simulink model "lwr_scheme_acc"  (R2024a)
settings: Solver=ode15s  StartTime=0.0  StopTime=10.0  FixedStep=0.1  RelTol=1e-3
undefined symbols (not defined in the file): X, Y, Z
libraries: sm_lib x73, nesl_utility x22, robotmaniplib x9, dspinverses x6
(part 2 of 2)

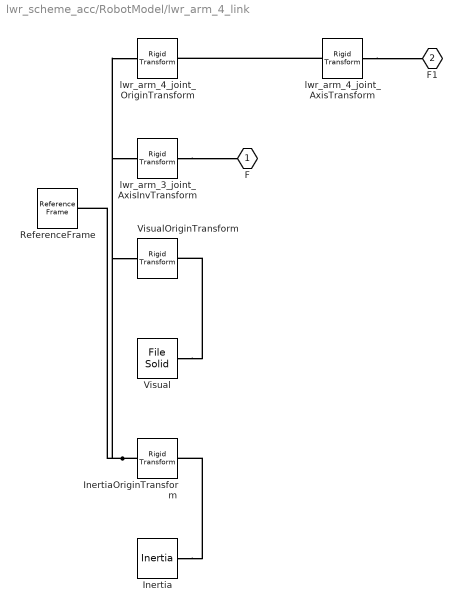
== system lwr_scheme_acc/RobotModel/lwr_arm_4_link ==
  Inertia : sm_lib/Body Elements/Inertia  InertiaType=Custom  Mass=2  MassUnits=kg  CenterOfMass=[0, 0, 0]  CenterOfMassUnits=m  MomentsOfInertia=[0.0136666666667, 0.0118666666667, 0.003000000000000001]  MomentsOfInertiaUnits=kg*m^2  ProductsOfInertia=[0, 0, 0]  ProductsOfInertiaUnits=kg*m^2  GraphicType=None  MarkerShape=Inertia  MarkerSize=20  GraphicVisPropType=SimpleVisualProperties  GraphicDiffuseColor=[0.5 0.5 0.5]  GraphicOpacity=1  GraphicSpecularColor=[0.5 0.5 0.5 1.0]  GraphicAmbientColor=[0.15 0.15 0.15 1.0]  GraphicEmissiveColor=[0.0 0.0 0.0 1.0]  GraphicShininess=75
  InertiaOriginTransform : sm_lib/Frames and Transforms/Rigid Transform  RotationMethod=RotationSequence  FollAlignAxisA=+X  BaseAlignAxisA=+Y  FollAlignAxisB=+Y  BaseAlignAxisB=+Z  RotationStandardAxis=+Z  RotationAngle=0  RotationAngleUnits=deg  RotationArbitraryAxis=[0 0 1]  RotationSequenceAxes=BaseAxes  RotationSequence=XYZ  RotationSequenceAngles=[0, 0, 0]  RotationSequenceAnglesUnits=rad  RotationMatrix=[1 0 0;0 1 0;0 0 1]  Quaternion=[1 0 0 0]  TranslationMethod=Cartesian  TranslationCartesianOffset=[0, 0.06, 0.07000000000000001]  TranslationCartesianOffsetUnits=m  TranslationStandardAxis=+Z  TranslationStandardOffset=0  TranslationStandardOffsetUnits=m  TranslationROffset=0  TranslationROffsetUnits=m  TranslationThetaOffset=0  TranslationThetaOffsetUnits=deg  TranslationZOffset=0  TranslationZOffsetUnits=m
  ReferenceFrame : sm_lib/Frames and Transforms/Reference Frame
  Visual : sm_lib/Body Elements/File Solid  ExtGeomFileName=/Users/salvatore/Desktop/Università/Development/Rob-HW/Damping-in-the-null-space-for-a-redundant-robot/robot_model/kuka-lwr-4plus/meshes/arm_segment_b.stl  UnitType=Custom  ExtGeomFileUnits=m  StepReaderType=HEX  ExportConvexHullGeometry=off  InertiaType=Custom  BasedOnType=DensityFromFile  Density=1000  DensityUnits=kg/m^3  Mass=0  MassUnits=kg  CenterOfMass=[0, 0, 0]  CenterOfMassUnits=m  MomentsOfInertia=[0, 0, 0]  MomentsOfInertiaUnits=kg*m^2  ProductsOfInertia=[0, 0, 0]  ProductsOfInertiaUnits=kg*m^2  GraphicType=FromGeometry  MarkerShape=Sphere  MarkerSize=10  GraphicVisPropType=SimpleVisualProperties  GraphicDiffuseColor=[1, 0.487, 0]  GraphicOpacity=1  GraphicSpecularColor=[0.5 0.5 0.5 1.0]  GraphicAmbientColor=[0.15 0.15 0.15 1.0]  GraphicEmissiveColor=[0.0 0.0 0.0 1.0]  GraphicShininess=75  DoExposeReferenceFrame=on  SerializedFrames=<Frames/>
  VisualOriginTransform : sm_lib/Frames and Transforms/Rigid Transform  RotationMethod=RotationSequence  FollAlignAxisA=+X  BaseAlignAxisA=+Y  FollAlignAxisB=+Y  BaseAlignAxisB=+Z  RotationStandardAxis=+Z  RotationAngle=0  RotationAngleUnits=deg  RotationArbitraryAxis=[0 0 1]  RotationSequenceAxes=BaseAxes  RotationSequence=XYZ  RotationSequenceAngles=[-3.141592653589793, -2.068231071102144e-13, 2.068231071102144e-13]  RotationSequenceAnglesUnits=rad  RotationMatrix=[1 0 0;0 1 0;0 0 1]  Quaternion=[1 0 0 0]  TranslationMethod=Cartesian  TranslationCartesianOffset=[0, 0, 0.2]  TranslationCartesianOffsetUnits=m  TranslationStandardAxis=+Z  TranslationStandardOffset=0  TranslationStandardOffsetUnits=m  TranslationROffset=0  TranslationROffsetUnits=m  TranslationThetaOffset=0  TranslationThetaOffsetUnits=deg  TranslationZOffset=0  TranslationZOffsetUnits=m
  lwr_arm_3_joint_AxisInvTransform : sm_lib/Frames and Transforms/Rigid Transform  RotationMethod=ArbitraryAxis  FollAlignAxisA=+X  BaseAlignAxisA=+Y  FollAlignAxisB=+Y  BaseAlignAxisB=+Z  RotationStandardAxis=+Z  RotationAngle=1.570796326794897  RotationAngleUnits=rad  RotationArbitraryAxis=[-1, 0, 0]  RotationSequenceAxes=FollowerAxes  RotationSequence=XYX  RotationSequenceAngles=[0 0 0]  RotationSequenceAnglesUnits=deg  RotationMatrix=[1 0 0;0 1 0;0 0 1]  Quaternion=[1 0 0 0]  TranslationMethod=Cartesian  TranslationCartesianOffset=[0, 0, 0]  TranslationCartesianOffsetUnits=m  TranslationStandardAxis=+Z  TranslationStandardOffset=0  TranslationStandardOffsetUnits=m  TranslationROffset=0  TranslationROffsetUnits=m  TranslationThetaOffset=0  TranslationThetaOffsetUnits=deg  TranslationZOffset=0  TranslationZOffsetUnits=m
  lwr_arm_4_joint_AxisTransform : sm_lib/Frames and Transforms/Rigid Transform  RotationMethod=ArbitraryAxis  FollAlignAxisA=+X  BaseAlignAxisA=+Y  FollAlignAxisB=+Y  BaseAlignAxisB=+Z  RotationStandardAxis=+Z  RotationAngle=0  RotationAngleUnits=rad  RotationArbitraryAxis=[1, 0, 0]  RotationSequenceAxes=FollowerAxes  RotationSequence=XYX  RotationSequenceAngles=[0 0 0]  RotationSequenceAnglesUnits=deg  RotationMatrix=[1 0 0;0 1 0;0 0 1]  Quaternion=[1 0 0 0]  TranslationMethod=Cartesian  TranslationCartesianOffset=[0, 0, 0]  TranslationCartesianOffsetUnits=m  TranslationStandardAxis=+Z  TranslationStandardOffset=0  TranslationStandardOffsetUnits=m  TranslationROffset=0  TranslationROffsetUnits=m  TranslationThetaOffset=0  TranslationThetaOffsetUnits=deg  TranslationZOffset=0  TranslationZOffsetUnits=m
  lwr_arm_4_joint_OriginTransform : sm_lib/Frames and Transforms/Rigid Transform  RotationMethod=RotationSequence  FollAlignAxisA=+X  BaseAlignAxisA=+Y  FollAlignAxisB=+Y  BaseAlignAxisB=+Z  RotationStandardAxis=+Z  RotationAngle=0  RotationAngleUnits=deg  RotationArbitraryAxis=[0 0 1]  RotationSequenceAxes=BaseAxes  RotationSequence=XYZ  RotationSequenceAngles=[0, 0, 0]  RotationSequenceAnglesUnits=rad  RotationMatrix=[1 0 0;0 1 0;0 0 1]  Quaternion=[1 0 0 0]  TranslationMethod=Cartesian  TranslationCartesianOffset=[0, 0, 0.2]  TranslationCartesianOffsetUnits=m  TranslationStandardAxis=+Z  TranslationStandardOffset=0  TranslationStandardOffsetUnits=m  TranslationROffset=0  TranslationROffsetUnits=m  TranslationThetaOffset=0  TranslationThetaOffsetUnits=deg  TranslationZOffset=0  TranslationZOffsetUnits=m
  F : PMIOPort  Side=Left
  F1 : PMIOPort  Port=2  Side=Right
  connections:
  Inertia/RConn1 -- InertiaOriginTransform/RConn1
  ReferenceFrame/RConn1 -- InertiaOriginTransform/LConn1 -- VisualOriginTransform/LConn1 -- lwr_arm_3_joint_AxisInvTransform/LConn1 -- lwr_arm_4_joint_OriginTransform/LConn1
  Visual/RConn1 -- VisualOriginTransform/RConn1
  lwr_arm_3_joint_AxisInvTransform/RConn1 -- F/RConn1
  lwr_arm_4_joint_AxisTransform/RConn1 -- F1/RConn1
  lwr_arm_4_joint_AxisTransform/LConn1 -- lwr_arm_4_joint_OriginTransform/RConn1

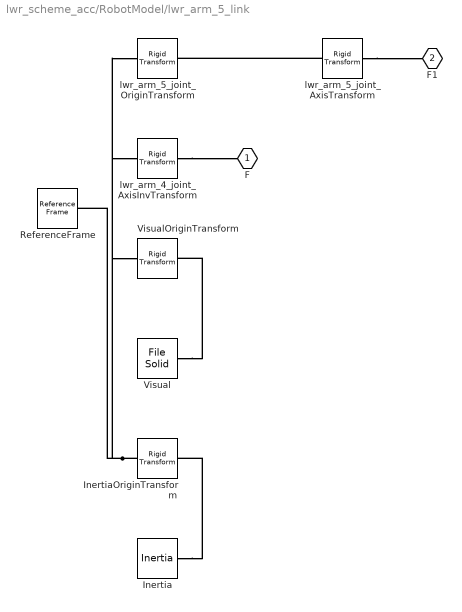
== system lwr_scheme_acc/RobotModel/lwr_arm_5_link ==
  Inertia : sm_lib/Body Elements/Inertia  InertiaType=Custom  Mass=2  MassUnits=kg  CenterOfMass=[0, 0, 0]  CenterOfMassUnits=m  MomentsOfInertia=[0.0126506666667, 0.0108506666667, 0.003]  MomentsOfInertiaUnits=kg*m^2  ProductsOfInertia=[0, 0, 0]  ProductsOfInertiaUnits=kg*m^2  GraphicType=None  MarkerShape=Inertia  MarkerSize=20  GraphicVisPropType=SimpleVisualProperties  GraphicDiffuseColor=[0.5 0.5 0.5]  GraphicOpacity=1  GraphicSpecularColor=[0.5 0.5 0.5 1.0]  GraphicAmbientColor=[0.15 0.15 0.15 1.0]  GraphicEmissiveColor=[0.0 0.0 0.0 1.0]  GraphicShininess=75
  InertiaOriginTransform : sm_lib/Frames and Transforms/Rigid Transform  RotationMethod=RotationSequence  FollAlignAxisA=+X  BaseAlignAxisA=+Y  FollAlignAxisB=+Y  BaseAlignAxisB=+Z  RotationStandardAxis=+Z  RotationAngle=0  RotationAngleUnits=deg  RotationArbitraryAxis=[0 0 1]  RotationSequenceAxes=BaseAxes  RotationSequence=XYZ  RotationSequenceAngles=[0, 0, 0]  RotationSequenceAnglesUnits=rad  RotationMatrix=[1 0 0;0 1 0;0 0 1]  Quaternion=[1 0 0 0]  TranslationMethod=Cartesian  TranslationCartesianOffset=[0, 0, 0.124]  TranslationCartesianOffsetUnits=m  TranslationStandardAxis=+Z  TranslationStandardOffset=0  TranslationStandardOffsetUnits=m  TranslationROffset=0  TranslationROffsetUnits=m  TranslationThetaOffset=0  TranslationThetaOffsetUnits=deg  TranslationZOffset=0  TranslationZOffsetUnits=m
  ReferenceFrame : sm_lib/Frames and Transforms/Reference Frame
  Visual : sm_lib/Body Elements/File Solid  ExtGeomFileName=/Users/salvatore/Desktop/Università/Development/Rob-HW/Damping-in-the-null-space-for-a-redundant-robot/robot_model/kuka-lwr-4plus/meshes/arm_segment_last.stl  UnitType=Custom  ExtGeomFileUnits=m  StepReaderType=HEX  ExportConvexHullGeometry=off  InertiaType=Custom  BasedOnType=DensityFromFile  Density=1000  DensityUnits=kg/m^3  Mass=0  MassUnits=kg  CenterOfMass=[0, 0, 0]  CenterOfMassUnits=m  MomentsOfInertia=[0, 0, 0]  MomentsOfInertiaUnits=kg*m^2  ProductsOfInertia=[0, 0, 0]  ProductsOfInertiaUnits=kg*m^2  GraphicType=FromGeometry  MarkerShape=Sphere  MarkerSize=10  GraphicVisPropType=SimpleVisualProperties  GraphicDiffuseColor=[1, 0.487, 0]  GraphicOpacity=1  GraphicSpecularColor=[0.5 0.5 0.5 1.0]  GraphicAmbientColor=[0.15 0.15 0.15 1.0]  GraphicEmissiveColor=[0.0 0.0 0.0 1.0]  GraphicShininess=75  DoExposeReferenceFrame=on  SerializedFrames=<Frames/>
  VisualOriginTransform : sm_lib/Frames and Transforms/Rigid Transform  RotationMethod=RotationSequence  FollAlignAxisA=+X  BaseAlignAxisA=+Y  FollAlignAxisB=+Y  BaseAlignAxisB=+Z  RotationStandardAxis=+Z  RotationAngle=0  RotationAngleUnits=deg  RotationArbitraryAxis=[0 0 1]  RotationSequenceAxes=BaseAxes  RotationSequence=XYZ  RotationSequenceAngles=[0, 0, -3.141592653589587]  RotationSequenceAnglesUnits=rad  RotationMatrix=[1 0 0;0 1 0;0 0 1]  Quaternion=[1 0 0 0]  TranslationMethod=Cartesian  TranslationCartesianOffset=[0, 0, 0]  TranslationCartesianOffsetUnits=m  TranslationStandardAxis=+Z  TranslationStandardOffset=0  TranslationStandardOffsetUnits=m  TranslationROffset=0  TranslationROffsetUnits=m  TranslationThetaOffset=0  TranslationThetaOffsetUnits=deg  TranslationZOffset=0  TranslationZOffsetUnits=m
  lwr_arm_4_joint_AxisInvTransform : sm_lib/Frames and Transforms/Rigid Transform  RotationMethod=ArbitraryAxis  FollAlignAxisA=+X  BaseAlignAxisA=+Y  FollAlignAxisB=+Y  BaseAlignAxisB=+Z  RotationStandardAxis=+Z  RotationAngle=0  RotationAngleUnits=rad  RotationArbitraryAxis=[1, 0, 0]  RotationSequenceAxes=FollowerAxes  RotationSequence=XYX  RotationSequenceAngles=[0 0 0]  RotationSequenceAnglesUnits=deg  RotationMatrix=[1 0 0;0 1 0;0 0 1]  Quaternion=[1 0 0 0]  TranslationMethod=Cartesian  TranslationCartesianOffset=[0, 0, 0]  TranslationCartesianOffsetUnits=m  TranslationStandardAxis=+Z  TranslationStandardOffset=0  TranslationStandardOffsetUnits=m  TranslationROffset=0  TranslationROffsetUnits=m  TranslationThetaOffset=0  TranslationThetaOffsetUnits=deg  TranslationZOffset=0  TranslationZOffsetUnits=m
  lwr_arm_5_joint_AxisTransform : sm_lib/Frames and Transforms/Rigid Transform  RotationMethod=ArbitraryAxis  FollAlignAxisA=+X  BaseAlignAxisA=+Y  FollAlignAxisB=+Y  BaseAlignAxisB=+Z  RotationStandardAxis=+Z  RotationAngle=1.570796326794897  RotationAngleUnits=rad  RotationArbitraryAxis=[1, 0, 0]  RotationSequenceAxes=FollowerAxes  RotationSequence=XYX  RotationSequenceAngles=[0 0 0]  RotationSequenceAnglesUnits=deg  RotationMatrix=[1 0 0;0 1 0;0 0 1]  Quaternion=[1 0 0 0]  TranslationMethod=Cartesian  TranslationCartesianOffset=[0, 0, 0]  TranslationCartesianOffsetUnits=m  TranslationStandardAxis=+Z  TranslationStandardOffset=0  TranslationStandardOffsetUnits=m  TranslationROffset=0  TranslationROffsetUnits=m  TranslationThetaOffset=0  TranslationThetaOffsetUnits=deg  TranslationZOffset=0  TranslationZOffsetUnits=m
  lwr_arm_5_joint_OriginTransform : sm_lib/Frames and Transforms/Rigid Transform  RotationMethod=RotationSequence  FollAlignAxisA=+X  BaseAlignAxisA=+Y  FollAlignAxisB=+Y  BaseAlignAxisB=+Z  RotationStandardAxis=+Z  RotationAngle=0  RotationAngleUnits=deg  RotationArbitraryAxis=[0 0 1]  RotationSequenceAxes=BaseAxes  RotationSequence=XYZ  RotationSequenceAngles=[0, 0, 0]  RotationSequenceAnglesUnits=rad  RotationMatrix=[1 0 0;0 1 0;0 0 1]  Quaternion=[1 0 0 0]  TranslationMethod=Cartesian  TranslationCartesianOffset=[0, 0, 0.19]  TranslationCartesianOffsetUnits=m  TranslationStandardAxis=+Z  TranslationStandardOffset=0  TranslationStandardOffsetUnits=m  TranslationROffset=0  TranslationROffsetUnits=m  TranslationThetaOffset=0  TranslationThetaOffsetUnits=deg  TranslationZOffset=0  TranslationZOffsetUnits=m
  F : PMIOPort  Side=Left
  F1 : PMIOPort  Port=2  Side=Right
  connections:
  Inertia/RConn1 -- InertiaOriginTransform/RConn1
  ReferenceFrame/RConn1 -- InertiaOriginTransform/LConn1 -- VisualOriginTransform/LConn1 -- lwr_arm_4_joint_AxisInvTransform/LConn1 -- lwr_arm_5_joint_OriginTransform/LConn1
  Visual/RConn1 -- VisualOriginTransform/RConn1
  lwr_arm_4_joint_AxisInvTransform/RConn1 -- F/RConn1
  lwr_arm_5_joint_AxisTransform/RConn1 -- F1/RConn1
  lwr_arm_5_joint_AxisTransform/LConn1 -- lwr_arm_5_joint_OriginTransform/RConn1

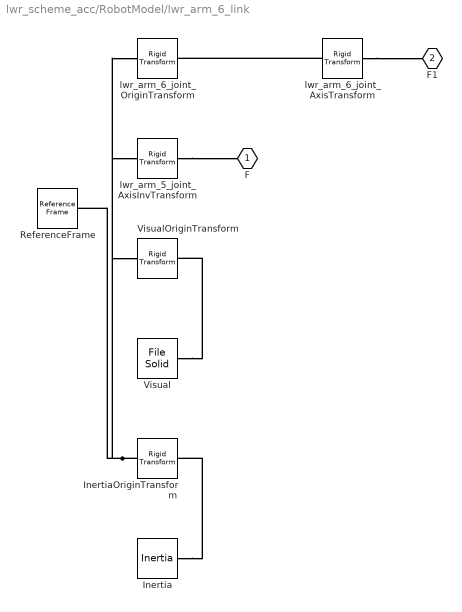
== system lwr_scheme_acc/RobotModel/lwr_arm_6_link ==
  Inertia : sm_lib/Body Elements/Inertia  InertiaType=Custom  Mass=1  MassUnits=kg  CenterOfMass=[0, 0, 0]  CenterOfMassUnits=m  MomentsOfInertia=[0.00260416666667, 0.00260416666667, 0.00260416666667]  MomentsOfInertiaUnits=kg*m^2  ProductsOfInertia=[0, 0, 0]  ProductsOfInertiaUnits=kg*m^2  GraphicType=None  MarkerShape=Inertia  MarkerSize=20  GraphicVisPropType=SimpleVisualProperties  GraphicDiffuseColor=[0.5 0.5 0.5]  GraphicOpacity=1  GraphicSpecularColor=[0.5 0.5 0.5 1.0]  GraphicAmbientColor=[0.15 0.15 0.15 1.0]  GraphicEmissiveColor=[0.0 0.0 0.0 1.0]  GraphicShininess=75
  InertiaOriginTransform : sm_lib/Frames and Transforms/Rigid Transform  RotationMethod=RotationSequence  FollAlignAxisA=+X  BaseAlignAxisA=+Y  FollAlignAxisB=+Y  BaseAlignAxisB=+Z  RotationStandardAxis=+Z  RotationAngle=0  RotationAngleUnits=deg  RotationArbitraryAxis=[0 0 1]  RotationSequenceAxes=BaseAxes  RotationSequence=XYZ  RotationSequenceAngles=[0, 0, 0]  RotationSequenceAnglesUnits=rad  RotationMatrix=[1 0 0;0 1 0;0 0 1]  Quaternion=[1 0 0 0]  TranslationMethod=Cartesian  TranslationCartesianOffset=[0, 0, 0]  TranslationCartesianOffsetUnits=m  TranslationStandardAxis=+Z  TranslationStandardOffset=0  TranslationStandardOffsetUnits=m  TranslationROffset=0  TranslationROffsetUnits=m  TranslationThetaOffset=0  TranslationThetaOffsetUnits=deg  TranslationZOffset=0  TranslationZOffsetUnits=m
  ReferenceFrame : sm_lib/Frames and Transforms/Reference Frame
  Visual : sm_lib/Body Elements/File Solid  ExtGeomFileName=/Users/salvatore/Desktop/Università/Development/Rob-HW/Damping-in-the-null-space-for-a-redundant-robot/robot_model/kuka-lwr-4plus/meshes/arm_wrist.stl  UnitType=Custom  ExtGeomFileUnits=m  StepReaderType=HEX  ExportConvexHullGeometry=off  InertiaType=Custom  BasedOnType=DensityFromFile  Density=1000  DensityUnits=kg/m^3  Mass=0  MassUnits=kg  CenterOfMass=[0, 0, 0]  CenterOfMassUnits=m  MomentsOfInertia=[0, 0, 0]  MomentsOfInertiaUnits=kg*m^2  ProductsOfInertia=[0, 0, 0]  ProductsOfInertiaUnits=kg*m^2  GraphicType=FromGeometry  MarkerShape=Sphere  MarkerSize=10  GraphicVisPropType=SimpleVisualProperties  GraphicDiffuseColor=[0.7, 0.7, 0.7]  GraphicOpacity=1  GraphicSpecularColor=[0.5 0.5 0.5 1.0]  GraphicAmbientColor=[0.15 0.15 0.15 1.0]  GraphicEmissiveColor=[0.0 0.0 0.0 1.0]  GraphicShininess=75  DoExposeReferenceFrame=on  SerializedFrames=<Frames/>
  VisualOriginTransform : sm_lib/Frames and Transforms/Rigid Transform  RotationMethod=RotationSequence  FollAlignAxisA=+X  BaseAlignAxisA=+Y  FollAlignAxisB=+Y  BaseAlignAxisB=+Z  RotationStandardAxis=+Z  RotationAngle=0  RotationAngleUnits=deg  RotationArbitraryAxis=[0 0 1]  RotationSequenceAxes=BaseAxes  RotationSequence=XYZ  RotationSequenceAngles=[0, 0, -3.141592653589587]  RotationSequenceAnglesUnits=rad  RotationMatrix=[1 0 0;0 1 0;0 0 1]  Quaternion=[1 0 0 0]  TranslationMethod=Cartesian  TranslationCartesianOffset=[0, 0, 0]  TranslationCartesianOffsetUnits=m  TranslationStandardAxis=+Z  TranslationStandardOffset=0  TranslationStandardOffsetUnits=m  TranslationROffset=0  TranslationROffsetUnits=m  TranslationThetaOffset=0  TranslationThetaOffsetUnits=deg  TranslationZOffset=0  TranslationZOffsetUnits=m
  lwr_arm_5_joint_AxisInvTransform : sm_lib/Frames and Transforms/Rigid Transform  RotationMethod=ArbitraryAxis  FollAlignAxisA=+X  BaseAlignAxisA=+Y  FollAlignAxisB=+Y  BaseAlignAxisB=+Z  RotationStandardAxis=+Z  RotationAngle=1.570796326794897  RotationAngleUnits=rad  RotationArbitraryAxis=[1, 0, 0]  RotationSequenceAxes=FollowerAxes  RotationSequence=XYX  RotationSequenceAngles=[0 0 0]  RotationSequenceAnglesUnits=deg  RotationMatrix=[1 0 0;0 1 0;0 0 1]  Quaternion=[1 0 0 0]  TranslationMethod=Cartesian  TranslationCartesianOffset=[0, 0, 0]  TranslationCartesianOffsetUnits=m  TranslationStandardAxis=+Z  TranslationStandardOffset=0  TranslationStandardOffsetUnits=m  TranslationROffset=0  TranslationROffsetUnits=m  TranslationThetaOffset=0  TranslationThetaOffsetUnits=deg  TranslationZOffset=0  TranslationZOffsetUnits=m
  lwr_arm_6_joint_AxisTransform : sm_lib/Frames and Transforms/Rigid Transform  RotationMethod=ArbitraryAxis  FollAlignAxisA=+X  BaseAlignAxisA=+Y  FollAlignAxisB=+Y  BaseAlignAxisB=+Z  RotationStandardAxis=+Z  RotationAngle=0  RotationAngleUnits=rad  RotationArbitraryAxis=[1, 0, 0]  RotationSequenceAxes=FollowerAxes  RotationSequence=XYX  RotationSequenceAngles=[0 0 0]  RotationSequenceAnglesUnits=deg  RotationMatrix=[1 0 0;0 1 0;0 0 1]  Quaternion=[1 0 0 0]  TranslationMethod=Cartesian  TranslationCartesianOffset=[0, 0, 0]  TranslationCartesianOffsetUnits=m  TranslationStandardAxis=+Z  TranslationStandardOffset=0  TranslationStandardOffsetUnits=m  TranslationROffset=0  TranslationROffsetUnits=m  TranslationThetaOffset=0  TranslationThetaOffsetUnits=deg  TranslationZOffset=0  TranslationZOffsetUnits=m
  lwr_arm_6_joint_OriginTransform : sm_lib/Frames and Transforms/Rigid Transform  RotationMethod=RotationSequence  FollAlignAxisA=+X  BaseAlignAxisA=+Y  FollAlignAxisB=+Y  BaseAlignAxisB=+Z  RotationStandardAxis=+Z  RotationAngle=0  RotationAngleUnits=deg  RotationArbitraryAxis=[0 0 1]  RotationSequenceAxes=BaseAxes  RotationSequence=XYZ  RotationSequenceAngles=[0, 0, 0]  RotationSequenceAnglesUnits=rad  RotationMatrix=[1 0 0;0 1 0;0 0 1]  Quaternion=[1 0 0 0]  TranslationMethod=Cartesian  TranslationCartesianOffset=[0, 0, 0.078]  TranslationCartesianOffsetUnits=m  TranslationStandardAxis=+Z  TranslationStandardOffset=0  TranslationStandardOffsetUnits=m  TranslationROffset=0  TranslationROffsetUnits=m  TranslationThetaOffset=0  TranslationThetaOffsetUnits=deg  TranslationZOffset=0  TranslationZOffsetUnits=m
  F : PMIOPort  Side=Left
  F1 : PMIOPort  Port=2  Side=Right
  connections:
  Inertia/RConn1 -- InertiaOriginTransform/RConn1
  ReferenceFrame/RConn1 -- InertiaOriginTransform/LConn1 -- VisualOriginTransform/LConn1 -- lwr_arm_5_joint_AxisInvTransform/LConn1 -- lwr_arm_6_joint_OriginTransform/LConn1
  Visual/RConn1 -- VisualOriginTransform/RConn1
  lwr_arm_5_joint_AxisInvTransform/RConn1 -- F/RConn1
  lwr_arm_6_joint_AxisTransform/RConn1 -- F1/RConn1
  lwr_arm_6_joint_AxisTransform/LConn1 -- lwr_arm_6_joint_OriginTransform/RConn1

== system lwr_scheme_acc/RobotModel/lwr_arm_7_link ==
  Inertia : sm_lib/Body Elements/Inertia  InertiaType=Custom  Mass=0.2  MassUnits=kg  CenterOfMass=[0, 0, 0]  CenterOfMassUnits=m  MomentsOfInertia=[6.66666666667e-05, 6.66666666667e-05, 0.00012]  MomentsOfInertiaUnits=kg*m^2  ProductsOfInertia=[0, 0, 0]  ProductsOfInertiaUnits=kg*m^2  GraphicType=None  MarkerShape=Inertia  MarkerSize=20  GraphicVisPropType=SimpleVisualProperties  GraphicDiffuseColor=[0.5 0.5 0.5]  GraphicOpacity=1  GraphicSpecularColor=[0.5 0.5 0.5 1.0]  GraphicAmbientColor=[0.15 0.15 0.15 1.0]  GraphicEmissiveColor=[0.0 0.0 0.0 1.0]  GraphicShininess=75
  InertiaOriginTransform : sm_lib/Frames and Transforms/Rigid Transform  RotationMethod=RotationSequence  FollAlignAxisA=+X  BaseAlignAxisA=+Y  FollAlignAxisB=+Y  BaseAlignAxisB=+Z  RotationStandardAxis=+Z  RotationAngle=0  RotationAngleUnits=deg  RotationArbitraryAxis=[0 0 1]  RotationSequenceAxes=BaseAxes  RotationSequence=XYZ  RotationSequenceAngles=[0, 0, 0]  RotationSequenceAnglesUnits=rad  RotationMatrix=[1 0 0;0 1 0;0 0 1]  Quaternion=[1 0 0 0]  TranslationMethod=Cartesian  TranslationCartesianOffset=[0, 0, 0]  TranslationCartesianOffsetUnits=m  TranslationStandardAxis=+Z  TranslationStandardOffset=0  TranslationStandardOffsetUnits=m  TranslationROffset=0  TranslationROffsetUnits=m  TranslationThetaOffset=0  TranslationThetaOffsetUnits=deg  TranslationZOffset=0  TranslationZOffsetUnits=m
  ReferenceFrame : sm_lib/Frames and Transforms/Reference Frame
  Visual : sm_lib/Body Elements/File Solid  ExtGeomFileName=/Users/salvatore/Desktop/Università/Development/Rob-HW/Damping-in-the-null-space-for-a-redundant-robot/robot_model/kuka-lwr-4plus/meshes/arm_flanche.stl  UnitType=Custom  ExtGeomFileUnits=m  StepReaderType=HEX  ExportConvexHullGeometry=off  InertiaType=Custom  BasedOnType=DensityFromFile  Density=1000  DensityUnits=kg/m^3  Mass=0  MassUnits=kg  CenterOfMass=[0, 0, 0]  CenterOfMassUnits=m  MomentsOfInertia=[0, 0, 0]  MomentsOfInertiaUnits=kg*m^2  ProductsOfInertia=[0, 0, 0]  ProductsOfInertiaUnits=kg*m^2  GraphicType=FromGeometry  MarkerShape=Sphere  MarkerSize=10  GraphicVisPropType=SimpleVisualProperties  GraphicDiffuseColor=[0.7, 0.7, 0.7]  GraphicOpacity=1  GraphicSpecularColor=[0.5 0.5 0.5 1.0]  GraphicAmbientColor=[0.15 0.15 0.15 1.0]  GraphicEmissiveColor=[0.0 0.0 0.0 1.0]  GraphicShininess=75  DoExposeReferenceFrame=on  SerializedFrames=<Frames/>
  VisualOriginTransform : sm_lib/Frames and Transforms/Rigid Transform  RotationMethod=RotationSequence  FollAlignAxisA=+X  BaseAlignAxisA=+Y  FollAlignAxisB=+Y  BaseAlignAxisB=+Z  RotationStandardAxis=+Z  RotationAngle=0  RotationAngleUnits=deg  RotationArbitraryAxis=[0 0 1]  RotationSequenceAxes=BaseAxes  RotationSequence=XYZ  RotationSequenceAngles=[0, 0, 0]  RotationSequenceAnglesUnits=rad  RotationMatrix=[1 0 0;0 1 0;0 0 1]  Quaternion=[1 0 0 0]  TranslationMethod=Cartesian  TranslationCartesianOffset=[0, 0, 0]  TranslationCartesianOffsetUnits=m  TranslationStandardAxis=+Z  TranslationStandardOffset=0  TranslationStandardOffsetUnits=m  TranslationROffset=0  TranslationROffsetUnits=m  TranslationThetaOffset=0  TranslationThetaOffsetUnits=deg  TranslationZOffset=0  TranslationZOffsetUnits=m
  lwr_arm_6_joint_AxisInvTransform : sm_lib/Frames and Transforms/Rigid Transform  RotationMethod=ArbitraryAxis  FollAlignAxisA=+X  BaseAlignAxisA=+Y  FollAlignAxisB=+Y  BaseAlignAxisB=+Z  RotationStandardAxis=+Z  RotationAngle=0  RotationAngleUnits=rad  RotationArbitraryAxis=[1, 0, 0]  RotationSequenceAxes=FollowerAxes  RotationSequence=XYX  RotationSequenceAngles=[0 0 0]  RotationSequenceAnglesUnits=deg  RotationMatrix=[1 0 0;0 1 0;0 0 1]  Quaternion=[1 0 0 0]  TranslationMethod=Cartesian  TranslationCartesianOffset=[0, 0, 0]  TranslationCartesianOffsetUnits=m  TranslationStandardAxis=+Z  TranslationStandardOffset=0  TranslationStandardOffsetUnits=m  TranslationROffset=0  TranslationROffsetUnits=m  TranslationThetaOffset=0  TranslationThetaOffsetUnits=deg  TranslationZOffset=0  TranslationZOffsetUnits=m
  F : PMIOPort  Side=Left
  connections:
  Inertia/RConn1 -- InertiaOriginTransform/RConn1
  ReferenceFrame/RConn1 -- InertiaOriginTransform/LConn1 -- VisualOriginTransform/LConn1 -- lwr_arm_6_joint_AxisInvTransform/LConn1
  Visual/RConn1 -- VisualOriginTransform/RConn1
  lwr_arm_6_joint_AxisInvTransform/RConn1 -- F/RConn1

== system lwr_scheme_acc/RobotModel/lwr_arm_base_link ==
  Inertia : sm_lib/Body Elements/Inertia  InertiaType=Custom  Mass=1.2  MassUnits=kg  CenterOfMass=[0, 0, 0]  CenterOfMassUnits=m  MomentsOfInertia=[0.00229, 0.00216, 0.00229]  MomentsOfInertiaUnits=kg*m^2  ProductsOfInertia=[0, 0, 0]  ProductsOfInertiaUnits=kg*m^2  GraphicType=None  MarkerShape=Inertia  MarkerSize=20  GraphicVisPropType=SimpleVisualProperties  GraphicDiffuseColor=[0.5 0.5 0.5]  GraphicOpacity=1  GraphicSpecularColor=[0.5 0.5 0.5 1.0]  GraphicAmbientColor=[0.15 0.15 0.15 1.0]  GraphicEmissiveColor=[0.0 0.0 0.0 1.0]  GraphicShininess=75
  InertiaOriginTransform : sm_lib/Frames and Transforms/Rigid Transform  RotationMethod=RotationSequence  FollAlignAxisA=+X  BaseAlignAxisA=+Y  FollAlignAxisB=+Y  BaseAlignAxisB=+Z  RotationStandardAxis=+Z  RotationAngle=0  RotationAngleUnits=deg  RotationArbitraryAxis=[0 0 1]  RotationSequenceAxes=BaseAxes  RotationSequence=XYZ  RotationSequenceAngles=[0, 0, 0]  RotationSequenceAnglesUnits=rad  RotationMatrix=[1 0 0;0 1 0;0 0 1]  Quaternion=[1 0 0 0]  TranslationMethod=Cartesian  TranslationCartesianOffset=[0, 0, 0.055]  TranslationCartesianOffsetUnits=m  TranslationStandardAxis=+Z  TranslationStandardOffset=0  TranslationStandardOffsetUnits=m  TranslationROffset=0  TranslationROffsetUnits=m  TranslationThetaOffset=0  TranslationThetaOffsetUnits=deg  TranslationZOffset=0  TranslationZOffsetUnits=m
  ReferenceFrame : sm_lib/Frames and Transforms/Reference Frame
  Visual : sm_lib/Body Elements/File Solid  ExtGeomFileName=/Users/salvatore/Desktop/Università/Development/Rob-HW/Damping-in-the-null-space-for-a-redundant-robot/robot_model/kuka-lwr-4plus/meshes/arm_base.stl  UnitType=Custom  ExtGeomFileUnits=m  StepReaderType=HEX  ExportConvexHullGeometry=off  InertiaType=Custom  BasedOnType=DensityFromFile  Density=1000  DensityUnits=kg/m^3  Mass=0  MassUnits=kg  CenterOfMass=[0, 0, 0]  CenterOfMassUnits=m  MomentsOfInertia=[0, 0, 0]  MomentsOfInertiaUnits=kg*m^2  ProductsOfInertia=[0, 0, 0]  ProductsOfInertiaUnits=kg*m^2  GraphicType=FromGeometry  MarkerShape=Sphere  MarkerSize=10  GraphicVisPropType=SimpleVisualProperties  GraphicDiffuseColor=[1, 0.487, 0]  GraphicOpacity=1  GraphicSpecularColor=[0.5 0.5 0.5 1.0]  GraphicAmbientColor=[0.15 0.15 0.15 1.0]  GraphicEmissiveColor=[0.0 0.0 0.0 1.0]  GraphicShininess=75  DoExposeReferenceFrame=on  SerializedFrames=<Frames/>
  VisualOriginTransform : sm_lib/Frames and Transforms/Rigid Transform  RotationMethod=RotationSequence  FollAlignAxisA=+X  BaseAlignAxisA=+Y  FollAlignAxisB=+Y  BaseAlignAxisB=+Z  RotationStandardAxis=+Z  RotationAngle=0  RotationAngleUnits=deg  RotationArbitraryAxis=[0 0 1]  RotationSequenceAxes=BaseAxes  RotationSequence=XYZ  RotationSequenceAngles=[0, 0, 0]  RotationSequenceAnglesUnits=rad  RotationMatrix=[1 0 0;0 1 0;0 0 1]  Quaternion=[1 0 0 0]  TranslationMethod=Cartesian  TranslationCartesianOffset=[0, 0, 0]  TranslationCartesianOffsetUnits=m  TranslationStandardAxis=+Z  TranslationStandardOffset=0  TranslationStandardOffsetUnits=m  TranslationROffset=0  TranslationROffsetUnits=m  TranslationThetaOffset=0  TranslationThetaOffsetUnits=deg  TranslationZOffset=0  TranslationZOffsetUnits=m
  lwr_arm_0_joint_AxisTransform : sm_lib/Frames and Transforms/Rigid Transform  RotationMethod=ArbitraryAxis  FollAlignAxisA=+X  BaseAlignAxisA=+Y  FollAlignAxisB=+Y  BaseAlignAxisB=+Z  RotationStandardAxis=+Z  RotationAngle=0  RotationAngleUnits=rad  RotationArbitraryAxis=[1, 0, 0]  RotationSequenceAxes=FollowerAxes  RotationSequence=XYX  RotationSequenceAngles=[0 0 0]  RotationSequenceAnglesUnits=deg  RotationMatrix=[1 0 0;0 1 0;0 0 1]  Quaternion=[1 0 0 0]  TranslationMethod=Cartesian  TranslationCartesianOffset=[0, 0, 0]  TranslationCartesianOffsetUnits=m  TranslationStandardAxis=+Z  TranslationStandardOffset=0  TranslationStandardOffsetUnits=m  TranslationROffset=0  TranslationROffsetUnits=m  TranslationThetaOffset=0  TranslationThetaOffsetUnits=deg  TranslationZOffset=0  TranslationZOffsetUnits=m
  lwr_arm_0_joint_OriginTransform : sm_lib/Frames and Transforms/Rigid Transform  RotationMethod=RotationSequence  FollAlignAxisA=+X  BaseAlignAxisA=+Y  FollAlignAxisB=+Y  BaseAlignAxisB=+Z  RotationStandardAxis=+Z  RotationAngle=0  RotationAngleUnits=deg  RotationArbitraryAxis=[0 0 1]  RotationSequenceAxes=BaseAxes  RotationSequence=XYZ  RotationSequenceAngles=[0, 0, 0]  RotationSequenceAnglesUnits=rad  RotationMatrix=[1 0 0;0 1 0;0 0 1]  Quaternion=[1 0 0 0]  TranslationMethod=Cartesian  TranslationCartesianOffset=[0, 0, 0.11]  TranslationCartesianOffsetUnits=m  TranslationStandardAxis=+Z  TranslationStandardOffset=0  TranslationStandardOffsetUnits=m  TranslationROffset=0  TranslationROffsetUnits=m  TranslationThetaOffset=0  TranslationThetaOffsetUnits=deg  TranslationZOffset=0  TranslationZOffsetUnits=m
  F : PMIOPort  Side=Left
  F1 : PMIOPort  Port=2  Side=Right
  connections:
  Inertia/RConn1 -- InertiaOriginTransform/RConn1
  ReferenceFrame/RConn1 -- InertiaOriginTransform/LConn1 -- VisualOriginTransform/LConn1 -- lwr_arm_0_joint_OriginTransform/LConn1 -- F/RConn1
  Visual/RConn1 -- VisualOriginTransform/RConn1
  lwr_arm_0_joint_AxisTransform/RConn1 -- F1/RConn1
  lwr_arm_0_joint_AxisTransform/LConn1 -- lwr_arm_0_joint_OriginTransform/RConn1

== system lwr_scheme_acc/RobotModel/world ==
  ReferenceFrame : sm_lib/Frames and Transforms/Reference Frame
  arm_world_joint_OriginTransform : sm_lib/Frames and Transforms/Rigid Transform  RotationMethod=RotationSequence  FollAlignAxisA=+X  BaseAlignAxisA=+Y  FollAlignAxisB=+Y  BaseAlignAxisB=+Z  RotationStandardAxis=+Z  RotationAngle=0  RotationAngleUnits=deg  RotationArbitraryAxis=[0 0 1]  RotationSequenceAxes=BaseAxes  RotationSequence=XYZ  RotationSequenceAngles=[0, 0, 0]  RotationSequenceAnglesUnits=rad  RotationMatrix=[1 0 0;0 1 0;0 0 1]  Quaternion=[1 0 0 0]  TranslationMethod=Cartesian  TranslationCartesianOffset=[0, 0, 0.01]  TranslationCartesianOffsetUnits=m  TranslationStandardAxis=+Z  TranslationStandardOffset=0  TranslationStandardOffsetUnits=m  TranslationROffset=0  TranslationROffsetUnits=m  TranslationThetaOffset=0  TranslationThetaOffsetUnits=deg  TranslationZOffset=0  TranslationZOffsetUnits=m
  F : PMIOPort  Side=Left
  F1 : PMIOPort  Port=2  Side=Right
  connections:
  arm_world_joint_OriginTransform/LConn1 -- ReferenceFrame/RConn1 -- F/RConn1
  arm_world_joint_OriginTransform/RConn1 -- F1/RConn1

== system lwr_scheme_acc/TorqueController/DLS ==
  matrix : Inport
  (lamda*I + mat*matT)^-1 : dspinverses/Pseudoinverse  wanterr=off  SimulateUsing=Interpreted execution
  Add : Sum
  Constant1 : Constant  Value=eye(3)
  Matrix Multiply : Product  Multiplication=Matrix(*)
  Transpose : Math  Operator=transpose
  Transpose1 : Math  Operator=transpose
  lamda : Gain  Gain=10
  mat*matT : Product  Multiplication=Matrix(*)
  inverse : Outport
  wires:
  matrix/1 -> Transpose/1, mat*matT/1, Transpose1/1
  Transpose1/1 -> mat*matT/2
  mat*matT/1 -> Add/2
  Add/1 -> (lamda*I + mat*matT)^-1/1
  (lamda*I + mat*matT)^-1/1 -> Matrix Multiply/2
  Matrix Multiply/1 -> inverse/1
  Constant1/1 -> lamda/1
  lamda/1 -> Add/1
  Transpose/1 -> Matrix Multiply/1

== system lwr_scheme_acc/invDynController/DLS1 ==
  matrix : Inport
  (lamda*I + mat*matT)^-1 : dspinverses/Pseudoinverse  wanterr=off  SimulateUsing=Interpreted execution
  Add : Sum
  Constant1 : Constant  Value=eye(3)
  Matrix Multiply : Product  Multiplication=Matrix(*)
  Transpose : Math  Operator=transpose
  Transpose1 : Math  Operator=transpose
  lamda : Gain  Gain=10
  mat*matT : Product  Multiplication=Matrix(*)
  inverse : Outport
  wires:
  matrix/1 -> Transpose/1, mat*matT/1, Transpose1/1
  Transpose1/1 -> mat*matT/2
  mat*matT/1 -> Add/2
  Add/1 -> (lamda*I + mat*matT)^-1/1
  (lamda*I + mat*matT)^-1/1 -> Matrix Multiply/2
  Matrix Multiply/1 -> inverse/1
  Constant1/1 -> lamda/1
  lamda/1 -> Add/1
  Transpose/1 -> Matrix Multiply/1

== system lwr_scheme_acc/simpler controller/DLS ==
  matrix : Inport
  (lamda*I + mat*matT)^-1 : dspinverses/Pseudoinverse  wanterr=off  SimulateUsing=Interpreted execution
  Add : Sum
  Constant1 : Constant  Value=eye(3)
  Matrix Multiply : Product  Multiplication=Matrix(*)
  Transpose : Math  Operator=transpose
  Transpose1 : Math  Operator=transpose
  lamda : Gain  Gain=10
  mat*matT : Product  Multiplication=Matrix(*)
  inverse : Outport
  wires:
  matrix/1 -> Transpose/1, mat*matT/1, Transpose1/1
  Transpose1/1 -> mat*matT/2
  mat*matT/1 -> Add/2
  Add/1 -> (lamda*I + mat*matT)^-1/1
  (lamda*I + mat*matT)^-1/1 -> Matrix Multiply/2
  Matrix Multiply/1 -> inverse/1
  Constant1/1 -> lamda/1
  lamda/1 -> Add/1
  Transpose/1 -> Matrix Multiply/1

== matlab function lwr_scheme_acc/invDynController/MATLAB Function5 ==
  data: t input; path_dot_vec output
function path_dot_vec = trajectory_dot(t)
radius = 0.5;
u_circle_plane = [1; 0; 0];  % must be unit vec and orth to v
v_circle_plane = [0; 1; 0];  % must be unit vec and orth to u
T = 10;  % trajectory duration in seconds
path_dot_vec = -u_circle_plane*radius*sin((t/T) * (2*pi))*((2*pi)/T) + v_circle_plane*radius*cos((t/T) * (2*pi))*((2*pi)/T);

== matlab function lwr_scheme_acc/invDynController/MATLAB Function6 ==
  data: configuration input; j output
function j = analytic_jacobian(configuration)
%ANALYTIC_JACOBIAN
%    J = ANALYTIC_JACOBIAN(Q1,Q2,Q3,Q4)

%    This function was generated by the Symbolic Math Toolbox version 24.1.
%    26-Jun-2024 11:14:32

q1 = configuration(1);
q2 = configuration(2);
q3 = configuration(3);
q4 = configuration(4);

t2 = cos(q1);
t3 = cos(q2);
t4 = cos(q3);
t5 = cos(q4);
t6 = sin(q1);
t7 = sin(q2);
t8 = sin(q3);
t9 = sin(q4);
t10 = t2.*t8;
t11 = t6.*t8;
t12 = t2.*t3.*t4;
t13 = t3.*t4.*t6;
t14 = -t12;
t15 = t10+t13;
t16 = t11+t14;
mt1 = [t6.*t7.*(2.0./5.0)-t9.*t15.*(3.9e+1./1.0e+2)+t5.*t6.*t7.*(3.9e+1./1.0e+2),t2.*t7.*(-2.0./5.0)-t9.*t16.*(3.9e+1./1.0e+2)-t2.*t5.*t7.*(3.9e+1./1.0e+2),0.0,t2.*t3.*(-2.0./5.0)-t2.*t3.*t5.*(3.9e+1./1.0e+2)-t2.*t4.*t7.*t9.*(3.9e+1./1.0e+2),t3.*t6.*(-2.0./5.0)-t3.*t5.*t6.*(3.9e+1./1.0e+2)-t4.*t6.*t7.*t9.*(3.9e+1./1.0e+2),t7.*(-2.0./5.0)-t5.*t7.*(3.9e+1./1.0e+2)+t3.*t4.*t9.*(3.9e+1./1.0e+2),t9.*(t4.*t6+t3.*t10).*(-3.9e+1./1.0e+2),t9.*(t2.*t4-t3.*t11).*(3.9e+1./1.0e+2),t7.*t8.*t9.*(-3.9e+1./1.0e+2)];
mt2 = [t5.*t16.*(-3.9e+1./1.0e+2)+t2.*t7.*t9.*(3.9e+1./1.0e+2),t5.*t15.*(3.9e+1./1.0e+2)+t6.*t7.*t9.*(3.9e+1./1.0e+2),t3.*t9.*(-3.9e+1./1.0e+2)+t4.*t5.*t7.*(3.9e+1./1.0e+2),0.0,0.0,0.0,0.0,0.0,0.0,0.0,0.0,0.0];
j = reshape([mt1,mt2],3,7);
end

== matlab function lwr_scheme_acc/TorqueController/MATLAB  funzione traiettoria ==
  data: t input; x output; R input; z0 input; y output; z output
function [x, y, z] = circular_trajectory(t, R, z0)
    x0=0.39;
    y0=0.39;
    x = x0+R * cos(t);
    y = y0+R * sin(t);
    z = z0;
end

== matlab function lwr_scheme_acc/TorqueController/MATLAB Function ==
  data: T input; f output
function f = poszione_robot(T)
f = T(1:3,4); % Posizione

end

== matlab function lwr_scheme_acc/TorqueController/MATLAB Function1 ==
  data: configuration input; j output
function j = analytic_jacobian(configuration)
%ANALYTIC_JACOBIAN
%    J = ANALYTIC_JACOBIAN(Q1,Q2,Q3,Q4)

%    This function was generated by the Symbolic Math Toolbox version 24.1.
%    26-Jun-2024 11:14:32

q1 = configuration(1);
q2 = configuration(2);
q3 = configuration(3);
q4 = configuration(4);

t2 = cos(q1);
t3 = cos(q2);
t4 = cos(q3);
t5 = cos(q4);
t6 = sin(q1);
t7 = sin(q2);
t8 = sin(q3);
t9 = sin(q4);
t10 = t2.*t8;
t11 = t6.*t8;
t12 = t2.*t3.*t4;
t13 = t3.*t4.*t6;
t14 = -t12;
t15 = t10+t13;
t16 = t11+t14;
mt1 = [t6.*t7.*(2.0./5.0)-t9.*t15.*(3.9e+1./1.0e+2)+t5.*t6.*t7.*(3.9e+1./1.0e+2),t2.*t7.*(-2.0./5.0)-t9.*t16.*(3.9e+1./1.0e+2)-t2.*t5.*t7.*(3.9e+1./1.0e+2),0.0,t2.*t3.*(-2.0./5.0)-t2.*t3.*t5.*(3.9e+1./1.0e+2)-t2.*t4.*t7.*t9.*(3.9e+1./1.0e+2),t3.*t6.*(-2.0./5.0)-t3.*t5.*t6.*(3.9e+1./1.0e+2)-t4.*t6.*t7.*t9.*(3.9e+1./1.0e+2),t7.*(-2.0./5.0)-t5.*t7.*(3.9e+1./1.0e+2)+t3.*t4.*t9.*(3.9e+1./1.0e+2),t9.*(t4.*t6+t3.*t10).*(-3.9e+1./1.0e+2),t9.*(t2.*t4-t3.*t11).*(3.9e+1./1.0e+2),t7.*t8.*t9.*(-3.9e+1./1.0e+2)];
mt2 = [t5.*t16.*(-3.9e+1./1.0e+2)+t2.*t7.*t9.*(3.9e+1./1.0e+2),t5.*t15.*(3.9e+1./1.0e+2)+t6.*t7.*t9.*(3.9e+1./1.0e+2),t3.*t9.*(-3.9e+1./1.0e+2)+t4.*t5.*t7.*(3.9e+1./1.0e+2),0.0,0.0,0.0,0.0,0.0,0.0,0.0,0.0,0.0];
j = reshape([mt1,mt2],3,7);
end

== matlab function lwr_scheme_acc/TorqueController/MATLAB  funzione traiettoria1 ==
  data: t input; xdot output; R input; ydot output; zdot output
function [xdot, ydot, zdot] = circular_trajectory_dot(t, R)
    xdot = -R * sin(t);
    ydot = R * cos(t);
    zdot = 0;
end

== matlab function lwr_scheme_acc/simpler controller/MATLAB Function1 ==
  data: configuration input; j output
function j = analytic_jacobian(configuration)
%ANALYTIC_JACOBIAN
%    J = ANALYTIC_JACOBIAN(Q1,Q2,Q3,Q4)

%    This function was generated by the Symbolic Math Toolbox version 24.1.
%    26-Jun-2024 11:14:32

q1 = configuration(1);
q2 = configuration(2);
q3 = configuration(3);
q4 = configuration(4);

t2 = cos(q1);
t3 = cos(q2);
t4 = cos(q3);
t5 = cos(q4);
t6 = sin(q1);
t7 = sin(q2);
t8 = sin(q3);
t9 = sin(q4);
t10 = t2.*t8;
t11 = t6.*t8;
t12 = t2.*t3.*t4;
t13 = t3.*t4.*t6;
t14 = -t12;
t15 = t10+t13;
t16 = t11+t14;
mt1 = [t6.*t7.*(2.0./5.0)-t9.*t15.*(3.9e+1./1.0e+2)+t5.*t6.*t7.*(3.9e+1./1.0e+2),t2.*t7.*(-2.0./5.0)-t9.*t16.*(3.9e+1./1.0e+2)-t2.*t5.*t7.*(3.9e+1./1.0e+2),0.0,t2.*t3.*(-2.0./5.0)-t2.*t3.*t5.*(3.9e+1./1.0e+2)-t2.*t4.*t7.*t9.*(3.9e+1./1.0e+2),t3.*t6.*(-2.0./5.0)-t3.*t5.*t6.*(3.9e+1./1.0e+2)-t4.*t6.*t7.*t9.*(3.9e+1./1.0e+2),t7.*(-2.0./5.0)-t5.*t7.*(3.9e+1./1.0e+2)+t3.*t4.*t9.*(3.9e+1./1.0e+2),t9.*(t4.*t6+t3.*t10).*(-3.9e+1./1.0e+2),t9.*(t2.*t4-t3.*t11).*(3.9e+1./1.0e+2),t7.*t8.*t9.*(-3.9e+1./1.0e+2)];
mt2 = [t5.*t16.*(-3.9e+1./1.0e+2)+t2.*t7.*t9.*(3.9e+1./1.0e+2),t5.*t15.*(3.9e+1./1.0e+2)+t6.*t7.*t9.*(3.9e+1./1.0e+2),t3.*t9.*(-3.9e+1./1.0e+2)+t4.*t5.*t7.*(3.9e+1./1.0e+2),0.0,0.0,0.0,0.0,0.0,0.0,0.0,0.0,0.0];
j = reshape([mt1,mt2],3,7);
end

== matlab function lwr_scheme_acc/TorqueController/MATLAB Function3 ==
  data: currJointPos input; j_dot output; currJointVel input
function j_dot = analytic_j_dot(currJointPos, currJointVel)
% function j_dot = analytic_j_dot(q1,q2,q3,q4,q_dot1,q_dot2,q_dot3,q_dot4)
%ANALYTIC_J_DOT
%    J_DOT = ANALYTIC_J_DOT(Q1,Q2,Q3,Q4,Q_DOT1,Q_DOT2,Q_DOT3,Q_DOT4)

%    This function was generated by the Symbolic Math Toolbox version 24.1.
%    26-Jun-2024 11:15:16

q1 = currJointPos(1);
q_dot1 = currJointVel(1);
q2 = currJointPos(2);
q_dot2 = currJointVel(2);
q3 = currJointPos(3);
q_dot3 = currJointVel(3);
q4 = currJointPos(4);
q_dot4 = currJointVel(4);

t2 = cos(q1);
t3 = cos(q2);
t4 = cos(q3);
t5 = cos(q4);
t6 = sin(q1);
t7 = sin(q2);
t8 = sin(q3);
t9 = sin(q4);
t10 = t2.*t8;
t11 = t6.*t8;
t12 = q_dot3.*t2.*t4;
t14 = q_dot3.*t4.*t6;
t16 = t2.*t3.*t4;
t17 = t3.*t4.*t6;
t20 = q_dot2.*t2.*t4.*t7;
t22 = q_dot2.*t4.*t6.*t7;
t13 = q_dot1.*t10;
t15 = q_dot1.*t11;
t18 = q_dot1.*t16;
t19 = q_dot1.*t17;
t21 = q_dot3.*t3.*t10;
t23 = q_dot3.*t3.*t11;
t24 = -t12;
t25 = -t16;
t27 = t10+t17;
t26 = -t18;
t28 = t11+t25;
t29 = t13+t14+t19+t20+t21;
t30 = t15+t22+t23+t24+t26;
mt1 = [t9.*t30.*(3.9e+1./1.0e+2)+q_dot1.*t2.*t7.*(2.0./5.0)+q_dot2.*t3.*t6.*(2.0./5.0)-q_dot4.*t5.*t27.*(3.9e+1./1.0e+2)+q_dot1.*t2.*t5.*t7.*(3.9e+1./1.0e+2)+q_dot2.*t3.*t5.*t6.*(3.9e+1./1.0e+2)-q_dot4.*t6.*t7.*t9.*(3.9e+1./1.0e+2),t9.*t29.*(-3.9e+1./1.0e+2)-q_dot2.*t2.*t3.*(2.0./5.0)+q_dot1.*t6.*t7.*(2.0./5.0)-q_dot4.*t5.*t28.*(3.9e+1./1.0e+2)-q_dot2.*t2.*t3.*t5.*(3.9e+1./1.0e+2)+q_dot1.*t5.*t6.*t7.*(3.9e+1./1.0e+2)+q_dot4.*t2.*t7.*t9.*(3.9e+1./1.0e+2),0.0];
mt2 = [q_dot1.*t3.*t6.*(2.0./5.0)+q_dot2.*t2.*t7.*(2.0./5.0)-q_dot2.*t9.*t16.*(3.9e+1./1.0e+2)+q_dot1.*t3.*t5.*t6.*(3.9e+1./1.0e+2)+q_dot2.*t2.*t5.*t7.*(3.9e+1./1.0e+2)+q_dot4.*t2.*t3.*t9.*(3.9e+1./1.0e+2)+q_dot3.*t7.*t9.*t10.*(3.9e+1./1.0e+2)-q_dot4.*t2.*t4.*t5.*t7.*(3.9e+1./1.0e+2)+q_dot1.*t4.*t6.*t7.*t9.*(3.9e+1./1.0e+2),q_dot1.*t2.*t3.*(-2.0./5.0)+q_dot2.*t6.*t7.*(2.0./5.0)-q_dot2.*t9.*t17.*(3.9e+1./1.0e+2)-q_dot1.*t2.*t3.*t5.*(3.9e+1./1.0e+2)+q_dot2.*t5.*t6.*t7.*(3.9e+1./1.0e+2)+q_dot4.*t3.*t6.*t9.*(3.9e+1./1.0e+2)+q_dot3.*t7.*t9.*t11.*(3.9e+1./1.0e+2)-q_dot1.*t2.*t4.*t7.*t9.*(3.9e+1./1.0e+2)-q_dot4.*t4.*t5.*t6.*t7.*(3.9e+1./1.0e+2)];
mt3 = [q_dot2.*t3.*(-2.0./5.0)-q_dot2.*t3.*t5.*(3.9e+1./1.0e+2)+q_dot4.*t7.*t9.*(3.9e+1./1.0e+2)+q_dot4.*t3.*t4.*t5.*(3.9e+1./1.0e+2)-q_dot2.*t4.*t7.*t9.*(3.9e+1./1.0e+2)-q_dot3.*t3.*t8.*t9.*(3.9e+1./1.0e+2),t9.*(q_dot3.*t11+t3.*t15+t3.*t24-q_dot1.*t2.*t4+q_dot2.*t7.*t10).*(3.9e+1./1.0e+2)-q_dot4.*t5.*(t4.*t6+t3.*t10).*(3.9e+1./1.0e+2),t9.*(q_dot3.*t10+t3.*t13+t3.*t14+q_dot1.*t4.*t6-q_dot2.*t7.*t11).*(-3.9e+1./1.0e+2)+q_dot4.*t5.*(t2.*t4-t3.*t11).*(3.9e+1./1.0e+2),q_dot2.*t3.*t8.*t9.*(-3.9e+1./1.0e+2)-q_dot3.*t4.*t7.*t9.*(3.9e+1./1.0e+2)-q_dot4.*t5.*t7.*t8.*(3.9e+1./1.0e+2)];
mt4 = [t5.*t29.*(-3.9e+1./1.0e+2)+q_dot4.*t9.*t28.*(3.9e+1./1.0e+2)+q_dot2.*t2.*t3.*t9.*(3.9e+1./1.0e+2)+q_dot4.*t2.*t5.*t7.*(3.9e+1./1.0e+2)-q_dot1.*t6.*t7.*t9.*(3.9e+1./1.0e+2),t5.*t30.*(-3.9e+1./1.0e+2)-q_dot4.*t9.*t27.*(3.9e+1./1.0e+2)+q_dot1.*t2.*t7.*t9.*(3.9e+1./1.0e+2)+q_dot2.*t3.*t6.*t9.*(3.9e+1./1.0e+2)+q_dot4.*t5.*t6.*t7.*(3.9e+1./1.0e+2),q_dot4.*t3.*t5.*(-3.9e+1./1.0e+2)+q_dot2.*t7.*t9.*(3.9e+1./1.0e+2)+q_dot2.*t3.*t4.*t5.*(3.9e+1./1.0e+2)-q_dot3.*t5.*t7.*t8.*(3.9e+1./1.0e+2)-q_dot4.*t4.*t7.*t9.*(3.9e+1./1.0e+2),0.0,0.0,0.0,0.0,0.0,0.0,0.0,0.0,0.0];
j_dot = reshape([mt1,mt2,mt3,mt4],3,7);
end

== matlab function lwr_scheme_acc/simpler controller/MATLAB Function ==
  data: t input; path_vec output
function path_vec = trajectory(t)
radius = 0.5;
circle_center = [0; 0; 0.4];
u_circle_plane = [1; 0; 0];  % must be unit vec and orth to v
v_circle_plane = [0; 1; 0];  % must be unit vec and orth to u
T = 10;  % trajectory duration in seconds
path_vec = circle_center + u_circle_plane*radius*cos((t/T) * (2*pi)) + v_circle_plane*radius*sin((t/T) * (2*pi));
end

== matlab function lwr_scheme_acc/simpler controller/MATLAB Function2 ==
  data: t input; path_dot_vec output
function path_dot_vec = trajectory_dot(t)
radius = 0.5;
u_circle_plane = [1; 0; 0];  % must be unit vec and orth to v
v_circle_plane = [0; 1; 0];  % must be unit vec and orth to u
T = 10;  % trajectory duration in seconds
path_dot_vec = -u_circle_plane*radius*sin((t/T) * (2*pi))*((2*pi)/T) + v_circle_plane*radius*cos((t/T) * (2*pi))*((2*pi)/T);
end

== matlab function lwr_scheme_acc/simpler controller/MATLAB Function3 ==
  data: T input; f output
function f = get_ee_pos(T)
f = T(1:3,4); % Posizione

end

== matlab function lwr_scheme_acc/simpler controller/MATLAB Function4 ==
  data: t input; path_dot_vec output
function path_dot_vec = trajectory_ddot(t)
radius = 0.5;
u_circle_plane = [1; 0; 0];  % must be unit vec and orth to v
v_circle_plane = [0; 1; 0];  % must be unit vec and orth to u
T = 10;  % trajectory duration in seconds
path_dot_vec = -u_circle_plane*radius*cos((t/T) * (2*pi))*((4*pi*pi)/(T*T)) - v_circle_plane*radius*sin((t/T) * (2*pi))*((4*pi*pi)/(T*T));
end

== matlab function lwr_scheme_acc/invDynController/MATLAB Function4 ==
  data: t input; path_hom_mat output
function path_hom_mat = trajectory(t)
radius = 0.5;
circle_center = [0; 0; 0.4];
u_circle_plane = [1; 0; 0];  % must be unit vec and orth to v
v_circle_plane = [0; 1; 0];  % must be unit vec and orth to u
T = 10;  % trajectory duration in seconds
path_vec = circle_center + u_circle_plane*radius*cos((t/T) * (2*pi)) + v_circle_plane*radius*sin((t/T) * (2*pi));

path_hom_mat = eye(4);
path_hom_mat(1:3, 4) = path_vec;
